simulink model "addNoise"  (R2015b)
settings: Solver=VariableStepAuto  StartTime=0.0  StopTime=10.0  RelTol=1e-3
undefined symbols (not defined in the file or in its folder): accelNoiseMax, accelNoiseMin, tstep
settings Model: Creator=araghunath  LastModifiedBy=araghunath

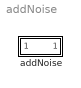
== system addNoise ==
  addNoise : Subsystem

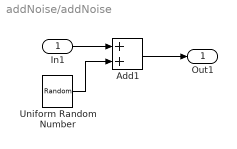
== system addNoise/addNoise ==
  In1 : Inport
  Add1 : Sum
  Uniform Random Number : UniformRandomNumber  Minimum=accelNoiseMin  Maximum=accelNoiseMax  SampleTime=tstep
  Out1 : Outport
  wires:
  Uniform Random Number/1 -> Add1/2
  In1/1 -> Add1/1
  Add1/1 -> Out1/1
